simulink model "xcoilSintonization"  (R2024a)
settings: Solver=VariableStepAuto  StartTime=0.0  StopTime=1000  RelTol=1e-3
undefined symbols (not defined in the file or in its folder): x
libraries: simulink x1
settings Model: Creator=workstation  LastModifiedBy=workstation
settings DataIOCC: SaveFormat=Array

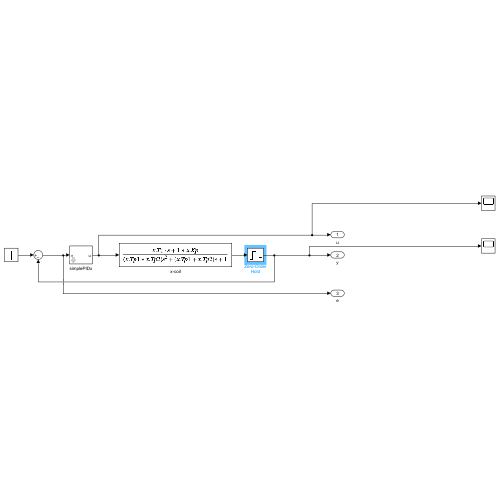
[thumbnail: Simulink's stored preview of the top-level diagram]
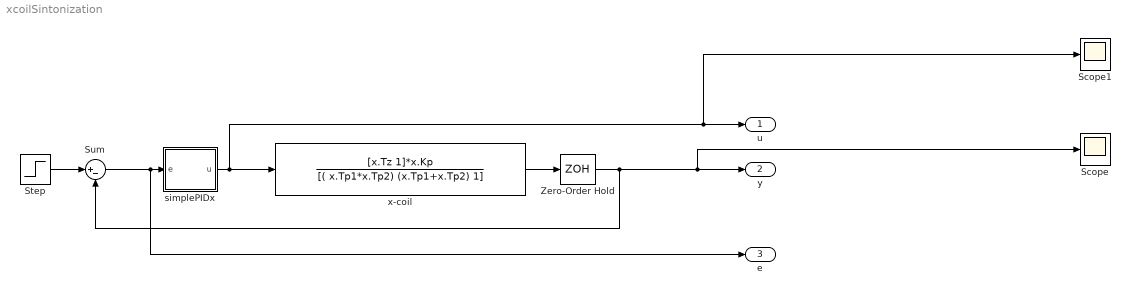
== system xcoilSintonization ==
  Scope : Scope
  Scope1 : Scope
  Step : Step  Time=0  SampleTime=0
  Sum : Sum  Inputs=|+-
  Zero-Order Hold : ZeroOrderHold
  simplePIDx : Subsystem  mask{Gain1=x.PID.Kd, Gain2=x.PID.Ki, Gain3=x.PID.Kp}
      mask prompts: Gain1 "kd:"; Gain2 "ki:"; Gain3 "kp:"
      mask TypeOptions Gain1: PID kd/Gain
      mask TypeOptions Gain2: PID ki/Gain
      mask TypeOptions Gain3: PID kp/Gain
  x-coil : TransferFcn  Numerator=[x.Tz 1]*x.Kp  Denominator=[( x.Tp1*x.Tp2) (x.Tp1+x.Tp2) 1]
  u : Outport
  y : Outport  Port=2
  e : Outport  Port=3
  wires:
  Sum/1 -> e/1, simplePIDx/1(e)
  Step/1 -> Sum/1
  simplePIDx/1(u) -> Scope1/1, u/1, x-coil/1
  x-coil/1 -> Zero-Order Hold/1
  Zero-Order Hold/1 -> Scope/1, y/1, Sum/2

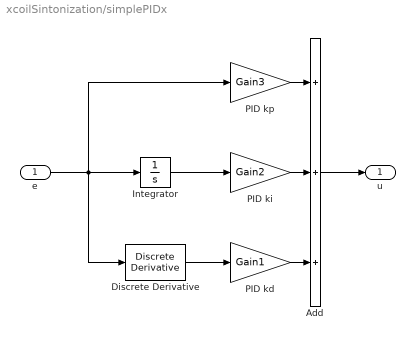
== system xcoilSintonization/simplePIDx ==
  e : Inport
  Add : Sum  Inputs=+++
  Discrete Derivative : simulink/Discrete/Discrete Derivative  gainval=1.0  ICPrevScaledInput=0.0  OutMin=[]  OutMax=[]  OutDataType=fixdt(1, 16)  OutScaling=2^-10  DoSatur=off
  Integrator : Integrator
  PID kd : Gain  Gain=Gain1
  PID ki : Gain  Gain=Gain2
  PID kp : Gain  Gain=Gain3
  u : Outport
  wires:
  Discrete Derivative/1 -> PID kd/1
  Add/1 -> u/1
  e/1 -> PID kp/1, Integrator/1, Discrete Derivative/1
  Integrator/1 -> PID ki/1
  PID ki/1 -> Add/2
  PID kd/1 -> Add/3
  PID kp/1 -> Add/1
